simulink model "play"  (R2023a)
settings: Solver=ode2  StartTime=0.0  StopTime=inf  FixedStep=1/30  RelTol=1e-3  EnableMultiTasking=on
StopFcn:
  | plot3(ee_pos.signals.values(1,:), ee_pos.signals.values(2,:), ee_pos.signals.values(3,:))
undefined symbols (not defined in the file): HIL, Host
libraries: quarc_library x8, simulink_extras x1, simulink x1
settings Model: SimulationMode=external  ExtModeTrigDuration=50000  Creator=msaravanan  LastModifiedBy=Mohit
settings SolverCC: PositivePriorityOrder=on
settings DataIOCC: SaveOutput=off  SaveTime=off  ReturnWorkspaceOutputs=off
settings RTWCC: Description=QUARC Win64 Target Using Toolchain  SystemTargetFile=quarc_win64.tlc  Toolchain=QUARC win64 | nmake (64-bit Windows)  BuildConfiguration=Faster Runs  GPUComputeCapability=5.0
settings STFCustomTargetCC: SystemTargetFile=quarc_win64.tlc
settings GRTTargetCC: ParMdlRefBuildCompliant=off  CompOptLevelCompliant=off  CombineOutputUpdateFcns=off  MatFileLogging=off  CPPClassGenCompliant=off  GRTInterface=on  ExtMode=on  ExtModeMexFile=quarc_comm

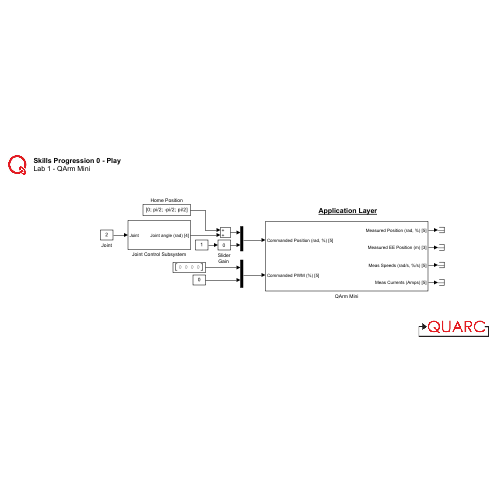
[thumbnail: Simulink's stored preview of the top-level diagram]
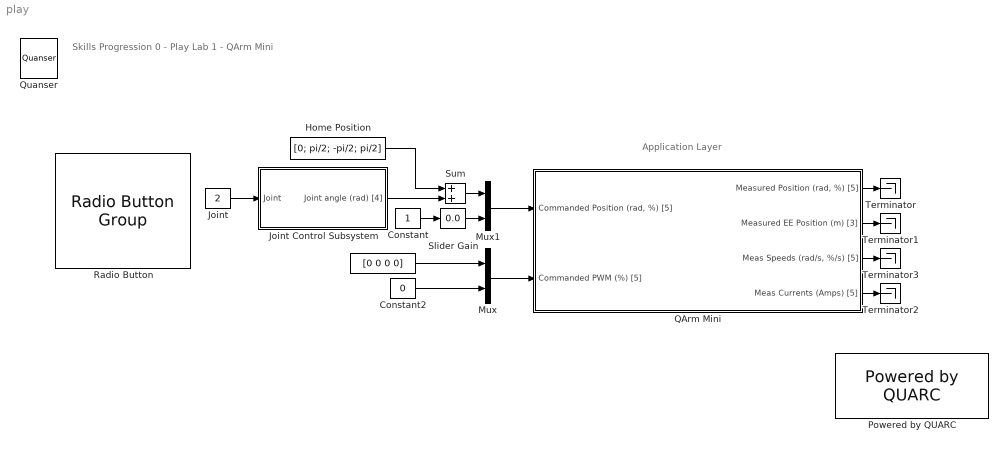
== system play ==
  note: Skills Progression 0 - Play
      | Lab 1 - QArm Mini
  note: Application Layer
  " " : Constant  Value=[0 0 0 0]
  Constant : Constant
  Constant2 : Constant  Value=0
  Home Position : Constant  Value=[0; pi/2; -pi/2; pi/2]  VectorParams1D=off
  Joint : Constant  Value=2
  Joint Control Subsystem : Subsystem
  Mux : Mux  Inputs=2
  Mux1 : Mux  Inputs=2
  Powered by QUARC : quarc_library/Logos/Powered by QUARC
  QArm Mini : Subsystem
  Quanser : quarc_library/Logos/Quanser
  Radio Button : RadioButtonGroup  SelectedLabel=Shoulder Joint  ButtonGroupName=Joint Selector
      settings: Values={{'Base Joint', 'Shoulder Joint', 'Elbow Joint', 'Wrist Joint'}, [1 2 3 4]}
  "Slider Gain " : simulink/Math Operations/Slider Gain  gain=0.0  low=0  high=1
  Sum : Sum
  Terminator{,1..3} (4 alike) : Terminator
  wires:
  Constant/1 -> "Slider Gain "/1
  QArm Mini/1("Measured Position (rad, %) [5]") -> Terminator/1
  QArm Mini/4(Meas Currents (Amps) [5]) -> Terminator2/1
  Mux/1 -> QArm Mini/2(Commanded PWM (%) [5])
  Constant2/1 -> Mux/2
  Mux1/1 -> QArm Mini/1("Commanded Position (rad, %) [5]")
  "Slider Gain "/1 -> Mux1/2
  QArm Mini/2(Measured EE Position (m) [3]) -> Terminator1/1
  Sum/1 -> Mux1/1
  Joint/1 -> Joint Control Subsystem/1(Joint)
  Joint Control Subsystem/1(Joint angle (rad) [4]) -> Sum/2
  Home Position/1 -> Sum/1
  QArm Mini/3("Meas Speeds (rad/s, %/s) [5]") -> Terminator3/1
  " "/1 -> Mux/1

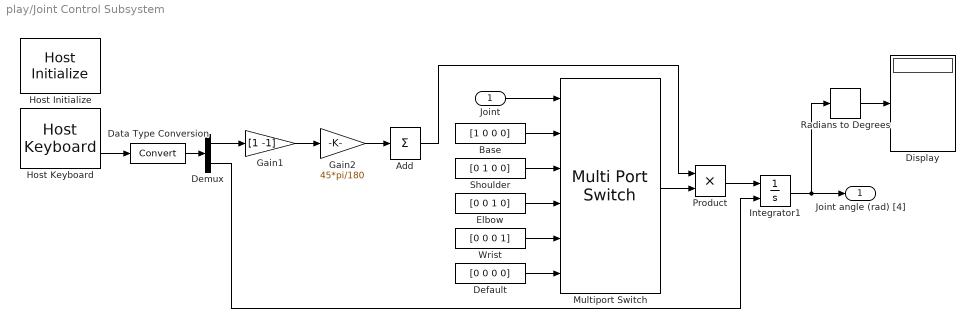
== system play/Joint Control Subsystem ==
  Joint : Inport
  Add : Sum  Inputs=1
  Base : Constant  Value=[1 0 0 0]
  Data Type Conversion : DataTypeConversion  SaturateOnIntegerOverflow=off  RndMeth=Floor
  Default : Constant  Value=[0 0 0 0]
  Demux : Demux  Outputs=2
  Display : Display
  Elbow : Constant  Value=[0 0 1 0]
  Gain1 : Gain  Gain=[1 -1]
  Gain2 : Gain  Gain=45*pi/180
  Host Initialize : quarc_library/Devices/Peripherals/Host/Host Initialize  object_name=Host-1  uri_source=Use external mode communications  uri=tcpip://localhost:18001  send_buffer_size=1000  receive_buffer_size=1000  thread_priority=0  run_client=on  use_window=off  window_position=[]  sample_time=qc_get_step_size  active=on
      settings: SourceProductName=QUARC Targets
  Host Keyboard : quarc_library/Devices/Peripherals/Host/Host Keyboard  object_name=Host-1  virtual_key="[38  40  32]"  sample_time=qc_get_step_size  enabled=on  debug_mode=off
      settings: SourceProductName=QUARC Targets
  Integrator1 : Integrator  ExternalReset=rising  LimitOutput=on  UpperSaturationLimit=[5*pi/4, pi/2, pi/2, pi/4]  LowerSaturationLimit=[-pi/2. -pi/2, -pi/4, -pi/2]
  Multiport Switch : MultiPortSwitch  Inputs=5  DiagnosticForDefault=Warning  SaturateOnIntegerOverflow=off  InputSameDT=off
  Product : Product
  Radians to Degrees : simulink_extras/Transformations/Radians to Degrees
  Shoulder : Constant  Value=[0 1 0 0]
  Wrist : Constant  Value=[0 0 0 1]
  Joint angle (rad) [4] : Outport
  wires:
  Host Keyboard/2 -> Data Type Conversion/1
  Data Type Conversion/1 -> Demux/1
  Gain2/1 -> Add/1
  Gain1/1 -> Gain2/1
  Default/1 -> Multiport Switch/6
  Joint/1 -> Multiport Switch/1
  Add/1 -> Product/1
  Multiport Switch/1 -> Product/2
  Shoulder/1 -> Multiport Switch/3
  Elbow/1 -> Multiport Switch/4
  Wrist/1 -> Multiport Switch/5
  Product/1 -> Integrator1/1
  Base/1 -> Multiport Switch/2
  Radians to Degrees/1 -> Display/1
  Demux/2 -> Integrator1/2
  Integrator1/1 -> Joint angle (rad) [4]/1, Radians to Degrees/1
  Demux/1 -> Gain1/1

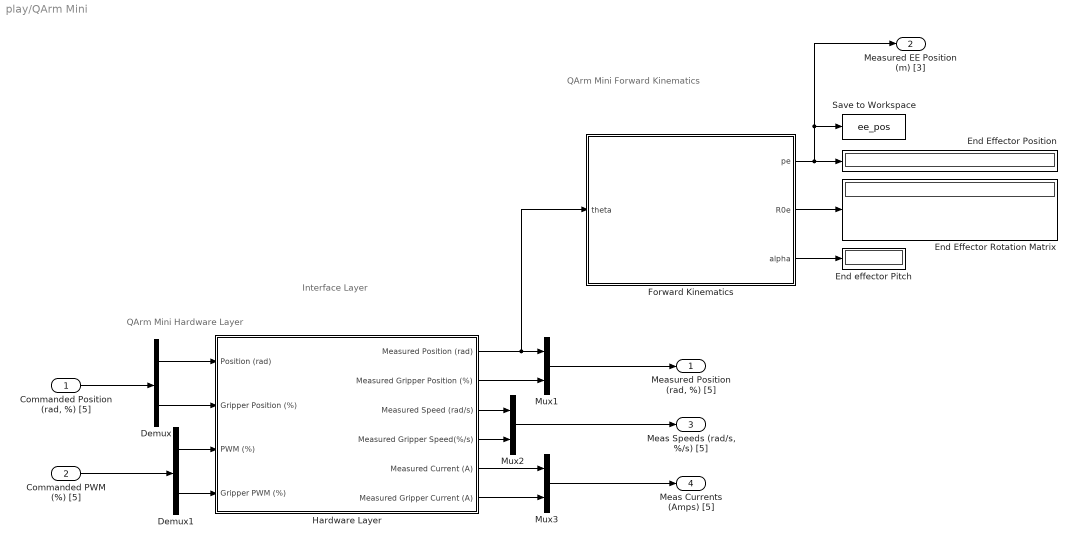
== system play/QArm Mini ==
  note: QArm Mini Forward Kinematics
  note: Interface Layer
  note: QArm Mini Hardware Layer
  "Commanded Position (rad, %) [5]" : Inport
  Commanded PWM (%) [5] : Inport  Port=2
  Demux : Demux  Outputs=[4 1]
  Demux1 : Demux  Outputs=[4 1]
  End Effector Position : Display
  End Effector Rotation Matrix : Display
  End effector Pitch : Display
  Forward Kinematics : MATLAB Function  TreatAsAtomicUnit=on
  Hardware Layer : Subsystem
  Mux1 : Mux  Inputs=2
  Mux2 : Mux  Inputs=2
  Mux3 : Mux  Inputs=2
  Save to Workspace : ToWorkspace  VariableName=ee_pos  SaveFormat=Structure With Time  SampleTime=-1
  "Measured Position (rad, %) [5]" : Outport
  Measured EE Position (m) [3] : Outport  Port=2
  "Meas Speeds (rad/s, %/s) [5]" : Outport  Port=3
  Meas Currents (Amps) [5] : Outport  Port=4
  wires:
  Demux/2 -> Hardware Layer/2(Gripper Position (%))
  Hardware Layer/1(Measured Position (rad)) -> Forward Kinematics/1(theta), Mux1/1
  Forward Kinematics/1(pe) -> Measured EE Position (m) [3]/1, Save to Workspace/1, End Effector Position/1
  Forward Kinematics/2(R0e) -> End Effector Rotation Matrix/1
  Forward Kinematics/3(alpha) -> End effector Pitch/1
  Demux1/2 -> Hardware Layer/4(Gripper PWM (%))
  Hardware Layer/2(Measured Gripper Position (%)) -> Mux1/2
  Hardware Layer/3(Measured Speed (rad/s)) -> Mux2/1
  Hardware Layer/4(Measured Gripper Speed(%/s)) -> Mux2/2
  Hardware Layer/5(Measured Current (A)) -> Mux3/1
  Hardware Layer/6(Measured Gripper Current (A)) -> Mux3/2
  Mux3/1 -> Meas Currents (Amps) [5]/1
  Mux2/1 -> "Meas Speeds (rad/s, %/s) [5]"/1
  Mux1/1 -> "Measured Position (rad, %) [5]"/1
  "Commanded Position (rad, %) [5]"/1 -> Demux/1
  Demux/1 -> Hardware Layer/1(Position (rad))
  Demux1/1 -> Hardware Layer/3(PWM (%))
  Commanded PWM (%) [5]/1 -> Demux1/1

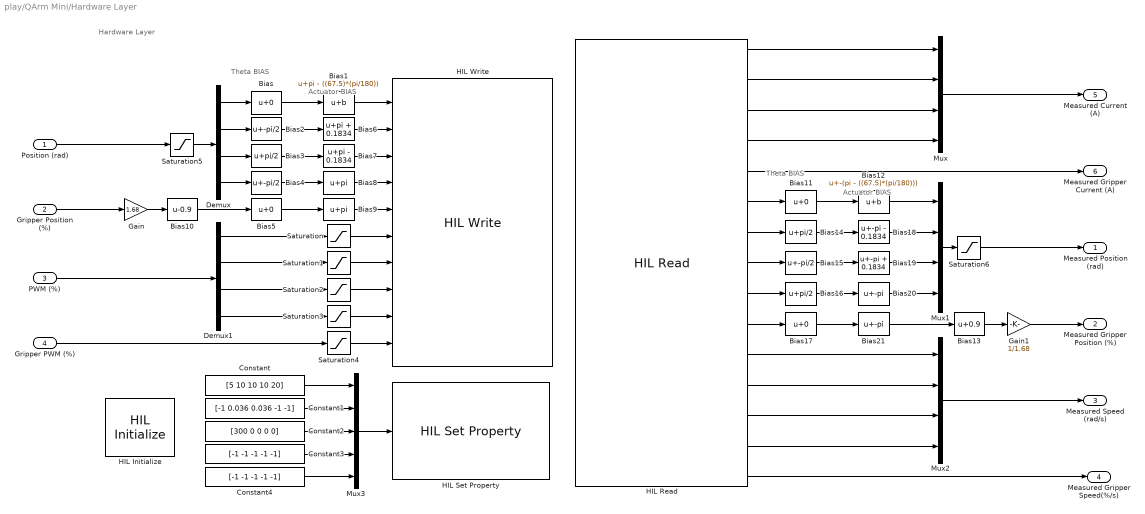
== system play/QArm Mini/Hardware Layer ==
  note: Hardware Layer
  note: Actuator BIAS
  note: Theta BIAS
  note: Actuator BIAS
  note: Theta BIAS
  Position (rad) : Inport
  Gripper Position (%) : Inport  Port=2
  PWM (%) : Inport  Port=3
  Gripper PWM (%) : Inport  Port=4
  Bias{,5,11,17} (4 alike) : Bias  SaturateOnIntegerOverflow=off
  Bias1 : Bias  Bias=pi - ((67.5)*(pi/180))  SaturateOnIntegerOverflow=off
  Bias10 : Bias  Bias=-0.9  SaturateOnIntegerOverflow=off
  Bias12 : Bias  Bias=-(pi - ((67.5)*(pi/180)))  SaturateOnIntegerOverflow=off
  Bias13 : Bias  Bias=0.9  SaturateOnIntegerOverflow=off
  Bias14 : Bias  Bias=pi/2  SaturateOnIntegerOverflow=off
  Bias15 : Bias  Bias=-pi/2  SaturateOnIntegerOverflow=off
  Bias16 : Bias  Bias=pi/2  SaturateOnIntegerOverflow=off
  Bias18 : Bias  Bias="-pi -  0.1834"  SaturateOnIntegerOverflow=off
  Bias19 : Bias  Bias="-pi +  0.1834"  SaturateOnIntegerOverflow=off
  Bias2 : Bias  Bias=-pi/2  SaturateOnIntegerOverflow=off
  Bias20 : Bias  Bias=-pi  SaturateOnIntegerOverflow=off
  Bias21 : Bias  Bias=-pi  SaturateOnIntegerOverflow=off
  Bias3 : Bias  Bias=pi/2  SaturateOnIntegerOverflow=off
  Bias4 : Bias  Bias=-pi/2  SaturateOnIntegerOverflow=off
  Bias6 : Bias  Bias=pi + 0.1834  SaturateOnIntegerOverflow=off
  Bias7 : Bias  Bias="pi -  0.1834"  SaturateOnIntegerOverflow=off
  Bias8 : Bias  Bias=pi  SaturateOnIntegerOverflow=off
  Bias9 : Bias  Bias=pi  SaturateOnIntegerOverflow=off
  Constant : Constant  Value=[5 10 10 10 20]
  Constant1 : Constant  Value=[-1 0.036 0.036 -1 -1]
  Constant2 : Constant  Value=[300 0 0 0 0]
  Constant3 : Constant  Value=[-1 -1 -1 -1 -1]
  Constant4 : Constant  Value=[-1 -1 -1 -1 -1]
  Demux : Demux
  Demux1 : Demux
  Gain : Gain  Gain=1.68
  Gain1 : Gain  Gain=1/1.68
  "HIL Initialize " : quarc_library/Data Acquisition/Generic/Configuration/HIL Initialize  object_name=HIL-1  board_type=qarm_mini  board_number=6  board_options=j0_mode=0;j1_mode=0;j2_mode=0;j3_mode=0;gripper_mode=0;j0_profile_velocity=6.2832;j0_profile_acceleration=6.2832;j1_profile_velocity=6.2832;j1_profile_acceleration=6.2832;j2_profile_velocity=6.2832;j2_profile_acceleration=6.2832;j3_profile_velocity=6.2832;j3_profile_acceleration=6.2832;gripper_profile_velocity=6.2832;gripper_profile_acceleration=6.2832;  exclusive=off  active=on  hardware_clocks=[]  clock_modes=[]  initial_clock_frequencies=[]  set_clock_params_at_start=off  set_clock_params_at_switch_in=off  set_clock_frequencies_at_start=off  set_clock_frequencies_at_switch_in=off  analog_input_channels=[0:4]  analog_input_configurations=[]  analog_input_maximums=[100 3.21 3.21 3.21 100]  analog_input_minimums=[-100 -3.21 -3.21 -3.21 -100]  set_analog_input_params_at_start=off  set_analog_input_params_at_switch_in=off  analog_output_channels=[]  analog_output_maximums=[]  analog_output_minimums=[]  initial_analog_outputs=[]  final_analog_outputs=[]  watchdog_analog_outputs=[]  set_analog_output_params_at_start=off  set_analog_output_params_at_switch_in=off  set_analog_outputs_at_start=off  set_analog_outputs_at_switch_in=off  set_analog_outputs_at_terminate=off  set_analog_outputs_at_switch_out=off  set_analog_outputs_on_watchdog=off  digital_input_channels=[]  digital_output_channels=[]  digital_output_configuration=[]  initial_digital_outputs=[]  final_digital_outputs=[]  watchdog_digital_outputs=[]  set_digital_output_params_at_start=off  set_digital_output_params_at_switch_in=off  set_digital_outputs_at_start=off  set_digital_outputs_at_switch_in=off  set_digital_outputs_at_terminate=off  set_digital_outputs_at_switch_out=off  set_digital_outputs_on_watchdog=off  encoder_channels=[]  quadrature=[]  encoder_filter_frequency=[]  initial_encoder_counts=[]  set_encoder_params_at_start=off  set_encoder_params_at_switch_in=off  set_encoder_counts_at_start=off  set_encoder_counts_at_switch_in=off  pwm_channels=[]  pwm_modes=[]  pwm_frequency=[]  pwm_configuration=[]  pwm_alignment=[]  pwm_polarity=[]  pwm_leading_deadband=[]  pwm_trailing_deadband=[]  initial_pwm_outputs=[]  final_pwm_outputs=[]  watchdog_pwm_outputs=[]  set_pwm_params_at_start=off  set_pwm_params_at_switch_in=off  set_pwm_outputs_at_start=off  set_pwm_outputs_at_switch_in=off  set_pwm_outputs_at_terminate=off  set_pwm_outputs_at_switch_out=off  set_pwm_outputs_on_watchdog=off  other_output_channels=[]  initial_other_outputs=[]  final_other_outputs=[]  watchdog_other_outputs=[]  set_other_outputs_at_start=off  set_other_outputs_at_switch_in=off  set_other_outputs_at_terminate=off  set_other_outputs_at_switch_out=off  set_other_outputs_on_watchdog=off
  HIL Read : quarc_library/Data Acquisition/Generic/Immediate I//O/HIL Read  object_name=HIL-1  analog_channels=[0:4]  encoder_channels=[]  digital_channels=[]  other_channels=[1000:1004 3000:3004]  sample_time=qc_get_step_size  active=on  vector_output=off  data_type_mode=Inherit via back propagation  encoder_data_type=double  digital_data_type=boolean
  HIL Set Property : quarc_library/Data Acquisition/Generic/Configuration/HIL Set Property  object_name=HIL-1  property_type=2  property_codes=[128:152]  property_source=2  property_value_num=0  set_at_start=on  sample_time=-1  active=off
      settings: AttributesFormatString=(%<object_name>)  SourceProductName=QUARC Targets
  HIL Write : quarc_library/Data Acquisition/Generic/Immediate I//O/HIL Write  object_name=HIL-1  analog_channels=[]  pwm_channels=[]  digital_channels=[]  other_channels=[1000:1004 11000:11004]  sample_time=-1  active=off  vector_input=off
  Mux : Mux
  Mux1 : Mux
  Mux2 : Mux
  Mux3 : Mux  Inputs=5
  Saturation{,1..4} (5 alike) : Saturate
  Saturation5 : Saturate  UpperLimit=[5*pi/4, pi, 0, 3*pi/4]'  LowerLimit=[-pi/2. 0, -3*pi/4, 0]'
  Saturation6 : Saturate  UpperLimit=[5*pi/4, pi, 0, 3*pi/4]'  LowerLimit=[-pi/2. 0, -3*pi/4, 0]'
  Measured Position (rad) : Outport
  Measured Gripper Position (%) : Outport  Port=2
  Measured Speed (rad/s) : Outport  Port=3
  Measured Gripper Speed(%/s) : Outport  Port=4
  Measured Current (A) : Outport  Port=5
  Measured Gripper Current (A) : Outport  Port=6
  wires:
  Position (rad)/1 -> Saturation5/1
  Demux/2 -> Bias2/1
  Demux/3 -> Bias3/1
  Demux/4 -> Bias4/1
  Bias/1 -> Bias1/1
  Bias1/1 -> HIL Write/1
  Bias2/1 -> Bias6/1
  Bias6/1 -> HIL Write/2
  Bias3/1 -> Bias7/1
  Bias7/1 -> HIL Write/3
  Bias4/1 -> Bias8/1
  Bias8/1 -> HIL Write/4
  Bias5/1 -> Bias9/1
  Bias9/1 -> HIL Write/5
  Gain/1 -> Bias10/1
  PWM (%)/1 -> Demux1/1
  Gripper PWM (%)/1 -> Saturation4/1
  Saturation/1 -> HIL Write/6
  Saturation1/1 -> HIL Write/7
  Saturation2/1 -> HIL Write/8
  Saturation3/1 -> HIL Write/9
  Saturation4/1 -> HIL Write/10
  HIL Read/1 -> Mux/1
  HIL Read/2 -> Mux/2
  HIL Read/3 -> Mux/3
  HIL Read/4 -> Mux/4
  Mux/1 -> Measured Current (A)/1
  HIL Read/5 -> Measured Gripper Current (A)/1
  Bias14/1 -> Bias18/1
  Bias15/1 -> Bias19/1
  Bias17/1 -> Bias21/1
  Bias11/1 -> Bias12/1
  Bias16/1 -> Bias20/1
  HIL Read/6 -> Bias11/1
  HIL Read/7 -> Bias14/1
  HIL Read/8 -> Bias15/1
  HIL Read/9 -> Bias16/1
  HIL Read/10 -> Bias17/1
  Bias21/1 -> Bias13/1
  Bias13/1 -> Gain1/1
  Gain1/1 -> Measured Gripper Position (%)/1
  Mux1/1 -> Saturation6/1
  HIL Read/11 -> Mux2/1
  HIL Read/12 -> Mux2/2
  HIL Read/13 -> Mux2/3
  HIL Read/14 -> Mux2/4
  Mux2/1 -> Measured Speed (rad/s)/1
  HIL Read/15 -> Measured Gripper Speed(%/s)/1
  Constant/1 -> Mux3/1
  Constant1/1 -> Mux3/2
  Constant2/1 -> Mux3/3
  Constant3/1 -> Mux3/4
  Constant4/1 -> Mux3/5
  Mux3/1 -> HIL Set Property/1
  Bias12/1 -> Mux1/1
  Bias18/1 -> Mux1/2
  Bias19/1 -> Mux1/3
  Bias20/1 -> Mux1/4
  Demux1/1 -> Saturation/1
  Demux1/2 -> Saturation1/1
  Demux1/3 -> Saturation2/1
  Demux1/4 -> Saturation3/1
  Demux/1 -> Bias/1
  Saturation5/1 -> Demux/1
  Saturation6/1 -> Measured Position (rad)/1
  Gripper Position (%)/1 -> Gain/1
  Bias10/1 -> Bias5/1

== matlab function play/QArm Mini/Forward Kinematics ==
  data: theta input; pe output; R0e output; alpha output
function [pe, R0e, alpha] = qArmMiniForwardKinematics(theta)

%% QARM_MINI_FPK
% v 1.0 - 30th March 2025

% REFERENCE: 
% Chapter 3. Forward Kinematics
% Robot Dynamics and Control 
% Spong, Vidyasagar
% 1989

% INPUTS:
% theta   : Alternate joint angles vector 4 x 1

% OUTPUTS:
% pe      : End-effector frame {e} position vector expressed in base frame {0}
% R0e     : rotation matrix from end-effector frame {e} to base frame {0}

%% Manipulator parameters:
L1 = 0.1300;
L2 = 0.1240;
L3 = 0.0230;
L4 = 0.1240;
L5 = 0.1320;

%% Alternate parameters
l1 = L1;
l2 = sqrt(L2^2 + L3^2);
l3 = L4;
l4 = L5;

%% Transformation matrices for all frames:

% T{i-1}{i} = quanser_arm_DH(  a, alpha,  d,     theta );
        T01 = quanser_arm_DH(  0,  pi/2, l1,  theta(1) );
        T12 = quanser_arm_DH( l2,     0,  0,  theta(2) );
        T23 = quanser_arm_DH( l3,     0,  0,  theta(3) );
        T34 = quanser_arm_DH(  0,  pi/2,  0,  theta(4) );
        T4e = quanser_arm_DH(  0,     0, l4,         0 );
        
        T02 = T01*T12;
        T03 = T02*T23;
        T04 = T03*T34;
        T0e = T04*T4e;
        
%% Position of end-effector Transformation

% Extract the Position vector 
p1   = T01(1:3,4);
p2   = T02(1:3,4);
p3   = T03(1:3,4);
p4   = T04(1:3,4);
pe   = T0e(1:3,4);

% Extract the Rotation matrix
R01 = T01(1:3,1:3);
R02 = T02(1:3,1:3);
R03 = T03(1:3,1:3);
R04 = T04(1:3,1:3);
R0e = T0e(1:3,1:3);
alpha = theta(2) + theta(3) + theta(4) - pi/2;
end

function T = quanser_arm_DH(a,alpha,d,theta)

%% QUANSER_ARM_DH
% v 1.0 - 26th March 2019

% REFERENCE: 
% Chapter 3. Forward and Inverse Kinematics
% Robot Modeling and Control 
% Spong, Hutchinson, Vidyasagar
% 2006

% INPUTS:
% a       :   translation  : along : x_{i}   : from : z_{i-1} : to : z_{i}
% alpha   :      rotation  : about : x_{i}   : from : z_{i-1} : to : z_{i}
% d       :   translation  : along : z_{i-1} : from : x_{i-1} : to : x_{i}
% theta   :      rotation  : about : z_{i-1} : from : x_{i-1} : to : x_{i}
% NOTE: Standard DH Parameters

% OUTPUTS:
% T       : transformation                   : from :     {i} : to : {i-1}

%%
% Rotation Transformation about z axis by theta
T_R_z = [cos(theta) -sin(theta) 0 0;
         sin(theta)  cos(theta) 0 0;
                  0           0 1 0;
                  0           0 0 1];
     
% Translation Transformation along z axis by d
T_T_z = [1 0 0 0;
         0 1 0 0;
         0 0 1 d;
         0 0 0 1];

% Translation Transformation along x axis by a
T_T_x = [1 0 0 a;
         0 1 0 0;
         0 0 1 0;
         0 0 0 1];

% Rotation Transformation about x axis by alpha
T_R_x = [1          0           0 0;
         0 cos(alpha) -sin(alpha) 0;
         0 sin(alpha)  cos(alpha) 0;
         0          0           0 1];

% For a transformation FROM frame {i} TO frame {i-1}: A
T = T_R_z*T_T_z*T_T_x*T_R_x;

end
